simulink model "system_MW"  (R2023b)
settings: Solver=VariableStepAuto  StartTime=0.0  StopTime=0.3  MaxStep=1e-3  RelTol=1e-3  AbsTol=1e-3  EnableMultiTasking=on
values from neighbouring files (symbols this model uses):
  Ts = ts(k)    [example_MW.m]
  Un = 400    [example_MW.m]
undefined symbols (not defined in the file or in its folder): P
libraries: fl_lib x41, nesl_utility x27, ee_lib x19, eeGeneralControl x8
(part 2 of 2)

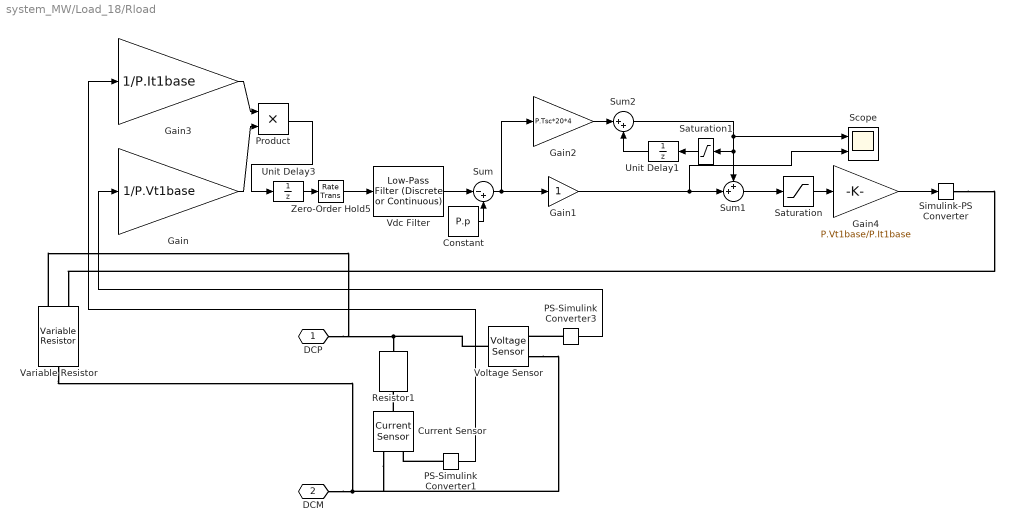
== system system_MW/Load_18/Rload ==
  Constant : Constant  Value=P.p
  Current Sensor : fl_lib/Electrical/Electrical Sensors/Current Sensor
  Gain : Gain  Gain=1/P.Vt1base
  Gain1 : Gain
  Gain2 : Gain  Gain=P.Tsc*20*4
  Gain3 : Gain  Gain=1/P.It1base
  Gain4 : Gain  Gain=P.Vt1base/P.It1base
  PS-Simulink Converter1 : nesl_utility/PS-Simulink Converter  PhysicalDomain=network_engine_domain  SubClassName=ps_output  LeftPortType=input  RightPortType=output  PseudoPeriodic=off  Frequencies=[]  VectorFormat=1-D array  Unit=1  AffineConversion=off
  PS-Simulink Converter3 : nesl_utility/PS-Simulink Converter  PhysicalDomain=network_engine_domain  SubClassName=ps_output  LeftPortType=input  RightPortType=output  PseudoPeriodic=off  Frequencies=[]  VectorFormat=1-D array  Unit=1  AffineConversion=off
  Product : Product
  Resistor1 : fl_lib/Electrical/Electrical Elements/Resistor  R=P.Un/P.In/P.p Ohm  i_specify=off  i_priority=None  i=0 A  i_nominal_specify=off  i_nominal_unit=A  i_nominal_value=1  v_specify=off  v_priority=None  v=0 V  v_nominal_specify=off  v_nominal_unit=V  v_nominal_value=1
  Saturation : Saturate  UpperLimit=10  LowerLimit=-10
  Saturation1 : Saturate  UpperLimit=10  LowerLimit=-10
  Scope : Scope  NumInputPorts=2
  Simulink-PS Converter : nesl_utility/Simulink-PS Converter  PhysicalDomain=network_engine_domain  SubClassName=ps_input  LeftPortType=input  RightPortType=output  PseudoPeriodic=off  Frequencies=[]  NoiseDistribution=none  NoiseParameters=[]  Unit=1  AffineConversion=off  FilteringAndDerivatives=provide  SimscapeFilterOrder=1  InputFilterTimeConstant=0.001  UdotUserProvided=0
  Sum : Sum  Inputs=|-+
  Sum1 : Sum  Inputs=++|
  Sum2 : Sum  Inputs=|++
  Unit Delay1 : UnitDelay  SampleTime=P.Tsc  HasFrameUpgradeWarning=on
  Unit Delay3 : UnitDelay  SampleTime=Ts  HasFrameUpgradeWarning=on
  Variable Resistor : fl_lib/Electrical/Electrical Elements/Variable Resistor  Rmin=0 Ohm  thermalEnable=false  thermal_mass=1 J/K  i_specify=off  i_priority=None  i=0 A  i_nominal_specify=off  i_nominal_unit=A  i_nominal_value=1  v_specify=off  v_priority=None  v=0 V  v_nominal_specify=off  v_nominal_unit=V  v_nominal_value=1  T_specify=off  T_priority=None  T=300 K  T_nominal_specify=off  T_nominal_unit=K  T_nominal_value=1
  Vdc Filter : eeGeneralControl/Low-Pass Filter (Discrete or Continuous)  K=1  T=1e-2  B=inf  A=-inf  init_option=Inherited from block input  x0=0  Ts=P.Tsc
  Voltage Sensor : fl_lib/Electrical/Electrical Sensors/Voltage Sensor
  Zero-Order Hold5 : RateTransition  OutPortSampleTime=P.Tsc
  DCP : PMIOPort  Side=Left
  DCM : PMIOPort  Port=2  Side=Left
  wires:
  Zero-Order Hold5/1 -> Vdc Filter/1
  PS-Simulink Converter3/1 -> Gain/1
  Unit Delay3/1 -> Zero-Order Hold5/1
  Vdc Filter/1 -> Sum/1
  Gain/1 -> Product/2
  Constant/1 -> Sum/2
  Sum1/1 -> Saturation/1
  Sum/1 -> Gain2/1, Gain1/1
  Sum2/1 -> Saturation1/1, Sum1/1, Scope/1
  Gain1/1 -> Scope/2, Sum1/2
  Gain2/1 -> Sum2/1
  Unit Delay1/1 -> Sum2/2
  PS-Simulink Converter1/1 -> Gain3/1
  Gain3/1 -> Product/1
  Product/1 -> Unit Delay3/1
  Saturation/1 -> Gain4/1
  Saturation1/1 -> Unit Delay1/1
  Gain4/1 -> Simulink-PS Converter/1
  connections:
  Voltage Sensor/LConn1 -- Resistor1/LConn1 -- DCP/RConn1 -- Variable Resistor/LConn2
  Variable Resistor/RConn1 -- DCM/RConn1 -- Voltage Sensor/RConn2 -- Current Sensor/RConn2
  PS-Simulink Converter3/LConn1 -- Voltage Sensor/RConn1
  Simulink-PS Converter/RConn1 -- Variable Resistor/LConn1
  Current Sensor/LConn1 -- Resistor1/RConn1
  PS-Simulink Converter1/LConn1 -- Current Sensor/RConn1

== system system_MW/Load_18/Vdc ==
  Voltage Source : ee_lib/Sources/Voltage Source  dc_voltage=P.Udc V  ac_voltage=0 V  ac_shift=0 rad  ac_frequency=fn Hz  noise_mode=ee.enum.sources.noise.Disabled  PSD=0 V^2/Hz  sample_time=1e-3 s  repeatability=ee.enum.sources.repeatability.NotRepeatable  user_seed=0  auto_seed=1336658428  i_specify=off  i_priority=None  i=0 A  i_nominal_specify=off  i_nominal_unit=A  i_nominal_value=1  v_specify=off  v_priority=None  v=0 V  v_nominal_specify=off  v_nominal_unit=V  v_nominal_value=1
  DCP : PMIOPort  Side=Left
  DCM : PMIOPort  Port=2  Side=Left
  connections:
  DCP/RConn1 -- Voltage Source/LConn1
  DCM/RConn1 -- Voltage Source/RConn1

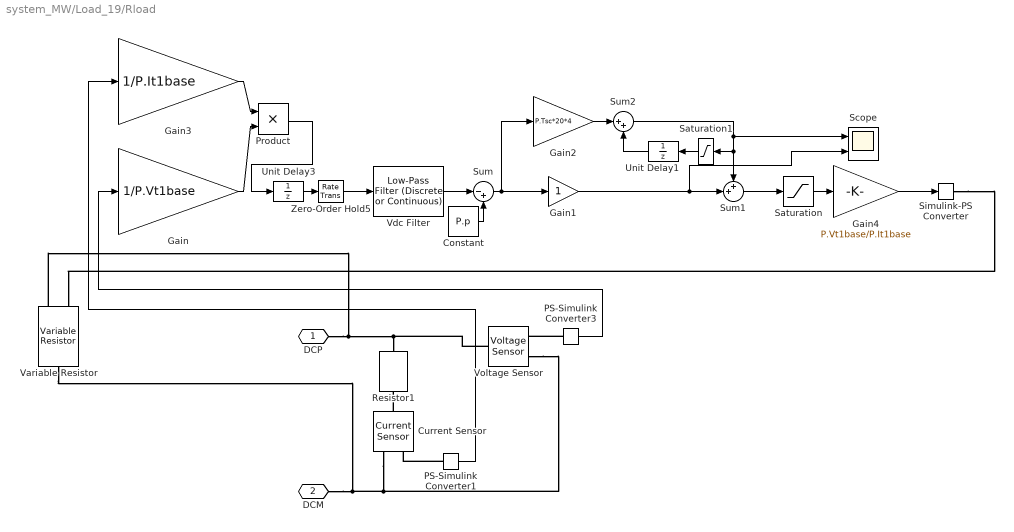
== system system_MW/Load_19/Rload ==
  Constant : Constant  Value=P.p
  Current Sensor : fl_lib/Electrical/Electrical Sensors/Current Sensor
  Gain : Gain  Gain=1/P.Vt1base
  Gain1 : Gain
  Gain2 : Gain  Gain=P.Tsc*20*4
  Gain3 : Gain  Gain=1/P.It1base
  Gain4 : Gain  Gain=P.Vt1base/P.It1base
  PS-Simulink Converter1 : nesl_utility/PS-Simulink Converter  PhysicalDomain=network_engine_domain  SubClassName=ps_output  LeftPortType=input  RightPortType=output  PseudoPeriodic=off  Frequencies=[]  VectorFormat=1-D array  Unit=1  AffineConversion=off
  PS-Simulink Converter3 : nesl_utility/PS-Simulink Converter  PhysicalDomain=network_engine_domain  SubClassName=ps_output  LeftPortType=input  RightPortType=output  PseudoPeriodic=off  Frequencies=[]  VectorFormat=1-D array  Unit=1  AffineConversion=off
  Product : Product
  Resistor1 : fl_lib/Electrical/Electrical Elements/Resistor  R=P.Un/P.In/P.p Ohm  i_specify=off  i_priority=None  i=0 A  i_nominal_specify=off  i_nominal_unit=A  i_nominal_value=1  v_specify=off  v_priority=None  v=0 V  v_nominal_specify=off  v_nominal_unit=V  v_nominal_value=1
  Saturation : Saturate  UpperLimit=10  LowerLimit=-10
  Saturation1 : Saturate  UpperLimit=10  LowerLimit=-10
  Scope : Scope  NumInputPorts=2
  Simulink-PS Converter : nesl_utility/Simulink-PS Converter  PhysicalDomain=network_engine_domain  SubClassName=ps_input  LeftPortType=input  RightPortType=output  PseudoPeriodic=off  Frequencies=[]  NoiseDistribution=none  NoiseParameters=[]  Unit=1  AffineConversion=off  FilteringAndDerivatives=provide  SimscapeFilterOrder=1  InputFilterTimeConstant=0.001  UdotUserProvided=0
  Sum : Sum  Inputs=|-+
  Sum1 : Sum  Inputs=++|
  Sum2 : Sum  Inputs=|++
  Unit Delay1 : UnitDelay  SampleTime=P.Tsc  HasFrameUpgradeWarning=on
  Unit Delay3 : UnitDelay  SampleTime=Ts  HasFrameUpgradeWarning=on
  Variable Resistor : fl_lib/Electrical/Electrical Elements/Variable Resistor  Rmin=0 Ohm  thermalEnable=false  thermal_mass=1 J/K  i_specify=off  i_priority=None  i=0 A  i_nominal_specify=off  i_nominal_unit=A  i_nominal_value=1  v_specify=off  v_priority=None  v=0 V  v_nominal_specify=off  v_nominal_unit=V  v_nominal_value=1  T_specify=off  T_priority=None  T=300 K  T_nominal_specify=off  T_nominal_unit=K  T_nominal_value=1
  Vdc Filter : eeGeneralControl/Low-Pass Filter (Discrete or Continuous)  K=1  T=1e-2  B=inf  A=-inf  init_option=Inherited from block input  x0=0  Ts=P.Tsc
  Voltage Sensor : fl_lib/Electrical/Electrical Sensors/Voltage Sensor
  Zero-Order Hold5 : RateTransition  OutPortSampleTime=P.Tsc
  DCP : PMIOPort  Side=Left
  DCM : PMIOPort  Port=2  Side=Left
  wires:
  Gain4/1 -> Simulink-PS Converter/1
  Saturation1/1 -> Unit Delay1/1
  Saturation/1 -> Gain4/1
  Product/1 -> Unit Delay3/1
  Gain3/1 -> Product/1
  PS-Simulink Converter1/1 -> Gain3/1
  Unit Delay1/1 -> Sum2/2
  Gain2/1 -> Sum2/1
  Gain1/1 -> Sum1/2, Scope/2
  Sum2/1 -> Scope/1, Sum1/1, Saturation1/1
  Sum/1 -> Gain1/1, Gain2/1
  Sum1/1 -> Saturation/1
  Constant/1 -> Sum/2
  Gain/1 -> Product/2
  Vdc Filter/1 -> Sum/1
  Unit Delay3/1 -> Zero-Order Hold5/1
  PS-Simulink Converter3/1 -> Gain/1
  Zero-Order Hold5/1 -> Vdc Filter/1
  connections:
  PS-Simulink Converter1/LConn1 -- Current Sensor/RConn1
  Current Sensor/LConn1 -- Resistor1/RConn1
  Simulink-PS Converter/RConn1 -- Variable Resistor/LConn1
  PS-Simulink Converter3/LConn1 -- Voltage Sensor/RConn1
  Current Sensor/RConn2 -- Voltage Sensor/RConn2 -- DCM/RConn1 -- Variable Resistor/RConn1
  Variable Resistor/LConn2 -- DCP/RConn1 -- Resistor1/LConn1 -- Voltage Sensor/LConn1

== system system_MW/Load_19/Vdc ==
  Voltage Source : ee_lib/Sources/Voltage Source  dc_voltage=P.Udc V  ac_voltage=0 V  ac_shift=0 rad  ac_frequency=fn Hz  noise_mode=ee.enum.sources.noise.Disabled  PSD=0 V^2/Hz  sample_time=1e-3 s  repeatability=ee.enum.sources.repeatability.NotRepeatable  user_seed=0  auto_seed=2270032532  i_specify=off  i_priority=None  i=0 A  i_nominal_specify=off  i_nominal_unit=A  i_nominal_value=1  v_specify=off  v_priority=None  v=0 V  v_nominal_specify=off  v_nominal_unit=V  v_nominal_value=1
  DCP : PMIOPort  Side=Left
  DCM : PMIOPort  Port=2  Side=Left
  connections:
  DCM/RConn1 -- Voltage Source/RConn1
  DCP/RConn1 -- Voltage Source/LConn1

== system system_MW/Load_20/Rload ==
  Resistor1 : fl_lib/Electrical/Electrical Elements/Resistor  R=P.Un/P.In/P.p Ohm  i_specify=off  i_priority=None  i=0 A  i_nominal_specify=off  i_nominal_unit=A  i_nominal_value=1  v_specify=off  v_priority=None  v=0 V  v_nominal_specify=off  v_nominal_unit=V  v_nominal_value=1
  DCP : PMIOPort  Side=Left
  DCM : PMIOPort  Port=2  Side=Left
  connections:
  DCP/RConn1 -- Resistor1/LConn1
  DCM/RConn1 -- Resistor1/RConn1

== system system_MW/Load_20/Vdc ==
  Voltage Source : ee_lib/Sources/Voltage Source  dc_voltage=P.Udc V  ac_voltage=0 V  ac_shift=0 rad  ac_frequency=fn Hz  noise_mode=ee.enum.sources.noise.Disabled  PSD=0 V^2/Hz  sample_time=1e-3 s  repeatability=ee.enum.sources.repeatability.NotRepeatable  user_seed=0  auto_seed=711455876  i_specify=off  i_priority=None  i=0 A  i_nominal_specify=off  i_nominal_unit=A  i_nominal_value=1  v_specify=off  v_priority=None  v=0 V  v_nominal_specify=off  v_nominal_unit=V  v_nominal_value=1
  DCP : PMIOPort  Side=Left
  DCM : PMIOPort  Port=2  Side=Left
  connections:
  DCP/RConn1 -- Voltage Source/LConn1
  DCM/RConn1 -- Voltage Source/RConn1

== system system_MW/Load_5/Rload ==
  Resistor1 : fl_lib/Electrical/Electrical Elements/Resistor  R=P.Un/P.In/P.p Ohm  i_specify=off  i_priority=None  i=0 A  i_nominal_specify=off  i_nominal_unit=A  i_nominal_value=1  v_specify=off  v_priority=None  v=0 V  v_nominal_specify=off  v_nominal_unit=V  v_nominal_value=1
  DCP : PMIOPort  Side=Left
  DCM : PMIOPort  Port=2  Side=Left
  connections:
  DCM/RConn1 -- Resistor1/RConn1
  DCP/RConn1 -- Resistor1/LConn1

== system system_MW/Load_5/Vdc ==
  Voltage Source : ee_lib/Sources/Voltage Source  dc_voltage=P.Udc V  ac_voltage=0 V  ac_shift=0 rad  ac_frequency=fn Hz  noise_mode=ee.enum.sources.noise.Disabled  PSD=0 V^2/Hz  sample_time=1e-3 s  repeatability=ee.enum.sources.repeatability.NotRepeatable  user_seed=0  auto_seed=2438775377  i_specify=off  i_priority=None  i=0 A  i_nominal_specify=off  i_nominal_unit=A  i_nominal_value=1  v_specify=off  v_priority=None  v=0 V  v_nominal_specify=off  v_nominal_unit=V  v_nominal_value=1
  DCP : PMIOPort  Side=Left
  DCM : PMIOPort  Port=2  Side=Left
  connections:
  DCM/RConn1 -- Voltage Source/RConn1
  DCP/RConn1 -- Voltage Source/LConn1

== system system_MW/Load_6/Rload ==
  Resistor1 : fl_lib/Electrical/Electrical Elements/Resistor  R=P.Un/P.In/P.p Ohm  i_specify=off  i_priority=None  i=0 A  i_nominal_specify=off  i_nominal_unit=A  i_nominal_value=1  v_specify=off  v_priority=None  v=0 V  v_nominal_specify=off  v_nominal_unit=V  v_nominal_value=1
  DCP : PMIOPort  Side=Left
  DCM : PMIOPort  Port=2  Side=Left
  connections:
  DCP/RConn1 -- Resistor1/LConn1
  DCM/RConn1 -- Resistor1/RConn1

== system system_MW/Load_6/Vdc ==
  Voltage Source : ee_lib/Sources/Voltage Source  dc_voltage=P.Udc V  ac_voltage=0 V  ac_shift=0 rad  ac_frequency=fn Hz  noise_mode=ee.enum.sources.noise.Disabled  PSD=0 V^2/Hz  sample_time=1e-3 s  repeatability=ee.enum.sources.repeatability.NotRepeatable  user_seed=0  auto_seed=325791693  i_specify=off  i_priority=None  i=0 A  i_nominal_specify=off  i_nominal_unit=A  i_nominal_value=1  v_specify=off  v_priority=None  v=0 V  v_nominal_specify=off  v_nominal_unit=V  v_nominal_value=1
  DCP : PMIOPort  Side=Left
  DCM : PMIOPort  Port=2  Side=Left
  connections:
  DCP/RConn1 -- Voltage Source/LConn1
  DCM/RConn1 -- Voltage Source/RConn1

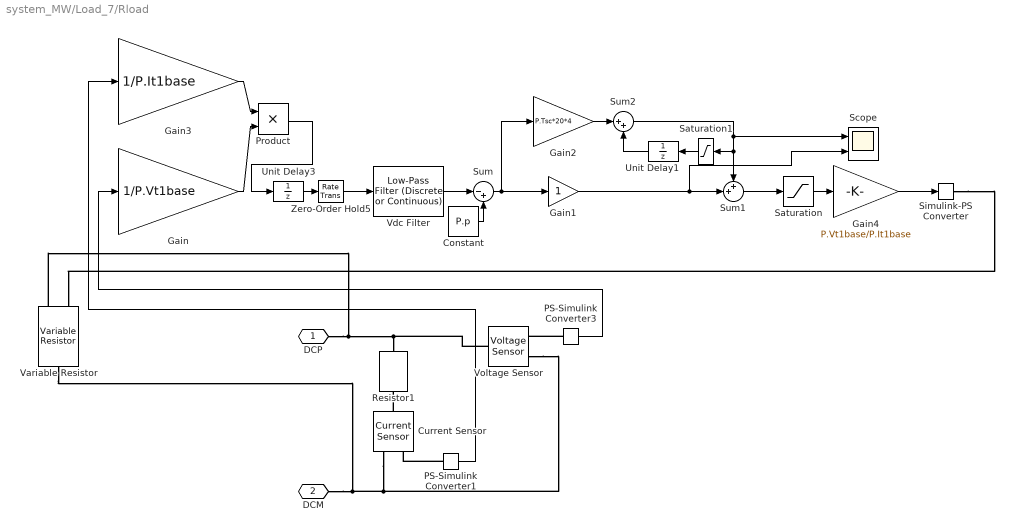
== system system_MW/Load_7/Rload ==
  Constant : Constant  Value=P.p
  Current Sensor : fl_lib/Electrical/Electrical Sensors/Current Sensor
  Gain : Gain  Gain=1/P.Vt1base
  Gain1 : Gain
  Gain2 : Gain  Gain=P.Tsc*20*4
  Gain3 : Gain  Gain=1/P.It1base
  Gain4 : Gain  Gain=P.Vt1base/P.It1base
  PS-Simulink Converter1 : nesl_utility/PS-Simulink Converter  PhysicalDomain=network_engine_domain  SubClassName=ps_output  LeftPortType=input  RightPortType=output  PseudoPeriodic=off  Frequencies=[]  VectorFormat=1-D array  Unit=1  AffineConversion=off
  PS-Simulink Converter3 : nesl_utility/PS-Simulink Converter  PhysicalDomain=network_engine_domain  SubClassName=ps_output  LeftPortType=input  RightPortType=output  PseudoPeriodic=off  Frequencies=[]  VectorFormat=1-D array  Unit=1  AffineConversion=off
  Product : Product
  Resistor1 : fl_lib/Electrical/Electrical Elements/Resistor  R=P.Un/P.In/P.p Ohm  i_specify=off  i_priority=None  i=0 A  i_nominal_specify=off  i_nominal_unit=A  i_nominal_value=1  v_specify=off  v_priority=None  v=0 V  v_nominal_specify=off  v_nominal_unit=V  v_nominal_value=1
  Saturation : Saturate  UpperLimit=10  LowerLimit=-10
  Saturation1 : Saturate  UpperLimit=10  LowerLimit=-10
  Scope : Scope  NumInputPorts=2
  Simulink-PS Converter : nesl_utility/Simulink-PS Converter  PhysicalDomain=network_engine_domain  SubClassName=ps_input  LeftPortType=input  RightPortType=output  PseudoPeriodic=off  Frequencies=[]  NoiseDistribution=none  NoiseParameters=[]  Unit=1  AffineConversion=off  FilteringAndDerivatives=provide  SimscapeFilterOrder=1  InputFilterTimeConstant=0.001  UdotUserProvided=0
  Sum : Sum  Inputs=|-+
  Sum1 : Sum  Inputs=++|
  Sum2 : Sum  Inputs=|++
  Unit Delay1 : UnitDelay  SampleTime=P.Tsc  HasFrameUpgradeWarning=on
  Unit Delay3 : UnitDelay  SampleTime=Ts  HasFrameUpgradeWarning=on
  Variable Resistor : fl_lib/Electrical/Electrical Elements/Variable Resistor  Rmin=0 Ohm  thermalEnable=false  thermal_mass=1 J/K  i_specify=off  i_priority=None  i=0 A  i_nominal_specify=off  i_nominal_unit=A  i_nominal_value=1  v_specify=off  v_priority=None  v=0 V  v_nominal_specify=off  v_nominal_unit=V  v_nominal_value=1  T_specify=off  T_priority=None  T=300 K  T_nominal_specify=off  T_nominal_unit=K  T_nominal_value=1
  Vdc Filter : eeGeneralControl/Low-Pass Filter (Discrete or Continuous)  K=1  T=1e-2  B=inf  A=-inf  init_option=Inherited from block input  x0=0  Ts=P.Tsc
  Voltage Sensor : fl_lib/Electrical/Electrical Sensors/Voltage Sensor
  Zero-Order Hold5 : RateTransition  OutPortSampleTime=P.Tsc
  DCP : PMIOPort  Side=Left
  DCM : PMIOPort  Port=2  Side=Left
  wires:
  Gain4/1 -> Simulink-PS Converter/1
  Saturation1/1 -> Unit Delay1/1
  Saturation/1 -> Gain4/1
  Product/1 -> Unit Delay3/1
  Gain3/1 -> Product/1
  PS-Simulink Converter1/1 -> Gain3/1
  Unit Delay1/1 -> Sum2/2
  Gain2/1 -> Sum2/1
  Gain1/1 -> Sum1/2, Scope/2
  Sum2/1 -> Scope/1, Sum1/1, Saturation1/1
  Sum/1 -> Gain1/1, Gain2/1
  Sum1/1 -> Saturation/1
  Constant/1 -> Sum/2
  Gain/1 -> Product/2
  Vdc Filter/1 -> Sum/1
  Unit Delay3/1 -> Zero-Order Hold5/1
  PS-Simulink Converter3/1 -> Gain/1
  Zero-Order Hold5/1 -> Vdc Filter/1
  connections:
  PS-Simulink Converter1/LConn1 -- Current Sensor/RConn1
  Current Sensor/LConn1 -- Resistor1/RConn1
  Simulink-PS Converter/RConn1 -- Variable Resistor/LConn1
  PS-Simulink Converter3/LConn1 -- Voltage Sensor/RConn1
  Current Sensor/RConn2 -- Voltage Sensor/RConn2 -- DCM/RConn1 -- Variable Resistor/RConn1
  Variable Resistor/LConn2 -- DCP/RConn1 -- Resistor1/LConn1 -- Voltage Sensor/LConn1

== system system_MW/Load_7/Vdc ==
  Voltage Source : ee_lib/Sources/Voltage Source  dc_voltage=P.Udc V  ac_voltage=0 V  ac_shift=0 rad  ac_frequency=fn Hz  noise_mode=ee.enum.sources.noise.Disabled  PSD=0 V^2/Hz  sample_time=1e-3 s  repeatability=ee.enum.sources.repeatability.NotRepeatable  user_seed=0  auto_seed=231713996  i_specify=off  i_priority=None  i=0 A  i_nominal_specify=off  i_nominal_unit=A  i_nominal_value=1  v_specify=off  v_priority=None  v=0 V  v_nominal_specify=off  v_nominal_unit=V  v_nominal_value=1
  DCP : PMIOPort  Side=Left
  DCM : PMIOPort  Port=2  Side=Left
  connections:
  DCM/RConn1 -- Voltage Source/RConn1
  DCP/RConn1 -- Voltage Source/LConn1

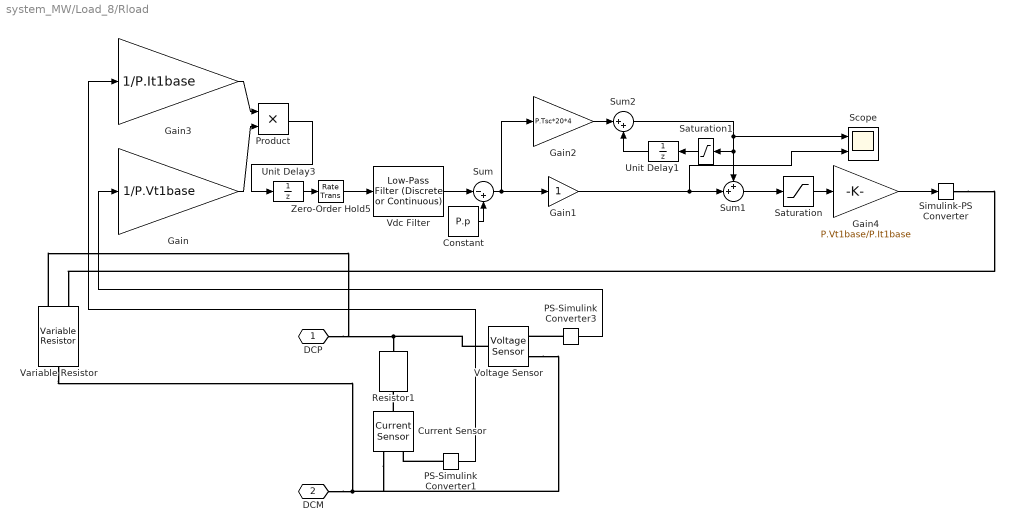
== system system_MW/Load_8/Rload ==
  Constant : Constant  Value=P.p
  Current Sensor : fl_lib/Electrical/Electrical Sensors/Current Sensor
  Gain : Gain  Gain=1/P.Vt1base
  Gain1 : Gain
  Gain2 : Gain  Gain=P.Tsc*20*4
  Gain3 : Gain  Gain=1/P.It1base
  Gain4 : Gain  Gain=P.Vt1base/P.It1base
  PS-Simulink Converter1 : nesl_utility/PS-Simulink Converter  PhysicalDomain=network_engine_domain  SubClassName=ps_output  LeftPortType=input  RightPortType=output  PseudoPeriodic=off  Frequencies=[]  VectorFormat=1-D array  Unit=1  AffineConversion=off
  PS-Simulink Converter3 : nesl_utility/PS-Simulink Converter  PhysicalDomain=network_engine_domain  SubClassName=ps_output  LeftPortType=input  RightPortType=output  PseudoPeriodic=off  Frequencies=[]  VectorFormat=1-D array  Unit=1  AffineConversion=off
  Product : Product
  Resistor1 : fl_lib/Electrical/Electrical Elements/Resistor  R=P.Un/P.In/P.p Ohm  i_specify=off  i_priority=None  i=0 A  i_nominal_specify=off  i_nominal_unit=A  i_nominal_value=1  v_specify=off  v_priority=None  v=0 V  v_nominal_specify=off  v_nominal_unit=V  v_nominal_value=1
  Saturation : Saturate  UpperLimit=10  LowerLimit=-10
  Saturation1 : Saturate  UpperLimit=10  LowerLimit=-10
  Scope : Scope  NumInputPorts=2
  Simulink-PS Converter : nesl_utility/Simulink-PS Converter  PhysicalDomain=network_engine_domain  SubClassName=ps_input  LeftPortType=input  RightPortType=output  PseudoPeriodic=off  Frequencies=[]  NoiseDistribution=none  NoiseParameters=[]  Unit=1  AffineConversion=off  FilteringAndDerivatives=provide  SimscapeFilterOrder=1  InputFilterTimeConstant=0.001  UdotUserProvided=0
  Sum : Sum  Inputs=|-+
  Sum1 : Sum  Inputs=++|
  Sum2 : Sum  Inputs=|++
  Unit Delay1 : UnitDelay  SampleTime=P.Tsc  HasFrameUpgradeWarning=on
  Unit Delay3 : UnitDelay  SampleTime=Ts  HasFrameUpgradeWarning=on
  Variable Resistor : fl_lib/Electrical/Electrical Elements/Variable Resistor  Rmin=0 Ohm  thermalEnable=false  thermal_mass=1 J/K  i_specify=off  i_priority=None  i=0 A  i_nominal_specify=off  i_nominal_unit=A  i_nominal_value=1  v_specify=off  v_priority=None  v=0 V  v_nominal_specify=off  v_nominal_unit=V  v_nominal_value=1  T_specify=off  T_priority=None  T=300 K  T_nominal_specify=off  T_nominal_unit=K  T_nominal_value=1
  Vdc Filter : eeGeneralControl/Low-Pass Filter (Discrete or Continuous)  K=1  T=1e-2  B=inf  A=-inf  init_option=Inherited from block input  x0=0  Ts=P.Tsc
  Voltage Sensor : fl_lib/Electrical/Electrical Sensors/Voltage Sensor
  Zero-Order Hold5 : RateTransition  OutPortSampleTime=P.Tsc
  DCP : PMIOPort  Side=Left
  DCM : PMIOPort  Port=2  Side=Left
  wires:
  Zero-Order Hold5/1 -> Vdc Filter/1
  PS-Simulink Converter3/1 -> Gain/1
  Unit Delay3/1 -> Zero-Order Hold5/1
  Vdc Filter/1 -> Sum/1
  Gain/1 -> Product/2
  Constant/1 -> Sum/2
  Sum1/1 -> Saturation/1
  Sum/1 -> Gain2/1, Gain1/1
  Sum2/1 -> Saturation1/1, Sum1/1, Scope/1
  Gain1/1 -> Scope/2, Sum1/2
  Gain2/1 -> Sum2/1
  Unit Delay1/1 -> Sum2/2
  PS-Simulink Converter1/1 -> Gain3/1
  Gain3/1 -> Product/1
  Product/1 -> Unit Delay3/1
  Saturation/1 -> Gain4/1
  Saturation1/1 -> Unit Delay1/1
  Gain4/1 -> Simulink-PS Converter/1
  connections:
  Voltage Sensor/LConn1 -- Resistor1/LConn1 -- DCP/RConn1 -- Variable Resistor/LConn2
  Variable Resistor/RConn1 -- DCM/RConn1 -- Voltage Sensor/RConn2 -- Current Sensor/RConn2
  PS-Simulink Converter3/LConn1 -- Voltage Sensor/RConn1
  Simulink-PS Converter/RConn1 -- Variable Resistor/LConn1
  Current Sensor/LConn1 -- Resistor1/RConn1
  PS-Simulink Converter1/LConn1 -- Current Sensor/RConn1

== system system_MW/Load_8/Vdc ==
  Voltage Source : ee_lib/Sources/Voltage Source  dc_voltage=P.Udc V  ac_voltage=0 V  ac_shift=0 rad  ac_frequency=fn Hz  noise_mode=ee.enum.sources.noise.Disabled  PSD=0 V^2/Hz  sample_time=1e-3 s  repeatability=ee.enum.sources.repeatability.NotRepeatable  user_seed=0  auto_seed=2279758131  i_specify=off  i_priority=None  i=0 A  i_nominal_specify=off  i_nominal_unit=A  i_nominal_value=1  v_specify=off  v_priority=None  v=0 V  v_nominal_specify=off  v_nominal_unit=V  v_nominal_value=1
  DCP : PMIOPort  Side=Left
  DCM : PMIOPort  Port=2  Side=Left
  connections:
  DCP/RConn1 -- Voltage Source/LConn1
  DCM/RConn1 -- Voltage Source/RConn1

== system system_MW/Load_9/Rload ==
  Resistor1 : fl_lib/Electrical/Electrical Elements/Resistor  R=P.Un/P.In/P.p Ohm  i_specify=off  i_priority=None  i=0 A  i_nominal_specify=off  i_nominal_unit=A  i_nominal_value=1  v_specify=off  v_priority=None  v=0 V  v_nominal_specify=off  v_nominal_unit=V  v_nominal_value=1
  DCP : PMIOPort  Side=Left
  DCM : PMIOPort  Port=2  Side=Left
  connections:
  DCP/RConn1 -- Resistor1/LConn1
  DCM/RConn1 -- Resistor1/RConn1

== system system_MW/Load_9/Vdc ==
  Voltage Source : ee_lib/Sources/Voltage Source  dc_voltage=P.Udc V  ac_voltage=0 V  ac_shift=0 rad  ac_frequency=fn Hz  noise_mode=ee.enum.sources.noise.Disabled  PSD=0 V^2/Hz  sample_time=1e-3 s  repeatability=ee.enum.sources.repeatability.NotRepeatable  user_seed=0  auto_seed=2443079021  i_specify=off  i_priority=None  i=0 A  i_nominal_specify=off  i_nominal_unit=A  i_nominal_value=1  v_specify=off  v_priority=None  v=0 V  v_nominal_specify=off  v_nominal_unit=V  v_nominal_value=1
  DCP : PMIOPort  Side=Left
  DCM : PMIOPort  Port=2  Side=Left
  connections:
  DCP/RConn1 -- Voltage Source/LConn1
  DCM/RConn1 -- Voltage Source/RConn1
